simulink model "UsvNuFLController"  (R2019b)
settings: Solver=ode3  StartTime=0.0  StopTime=Inf  FixedStep=0.01  RelTol=1e-3  EnableMultiTasking=on
undefined symbols (not defined in the file): Theta, X
libraries: robotlib x8, simulink x2
settings Model: Creator=The MathWorks, Inc.  LastModifiedBy=alex
settings DataIOCC: LimitDataPoints=on  SaveFormat=Array  ReturnWorkspaceOutputs=off
settings OptimizationCC: LifeSpan=Inf  MaxStackSize=64
settings DebuggingCC: SolverPrmCheckMsg=warning  AllowSymbolicDim=off  SFUnexpectedBacktrackingDiag=warning  SFNoUnconditionalDefaultTransitionDiag=warning  SFExecutionAtInitializationDiag=none  ArithmeticOperatorsInVariantConditions=warning
settings HardwareCC: ProdBitPerLong=64  ProdHWDeviceType=Intel->x86-64 (Linux 64)  TargetHWDeviceType=Generic->Unspecified (assume 32-bit Generic)  UseEmbeddedCoderFeatures=off
settings ModelReferenceCC: PropagateSignalLabelsOutOfModel=off
settings SFSimCC: SimUseLocalCustomCode=off  CustomCodeUndefinedFunction=UseInterfaceOnly
settings RTWCC: SystemTargetFile=ert.tlc  HardwareBoard=Robot Operating System (ROS)  TemplateMakefile=ert_default_tmf  RTWUseLocalCustomCode=off  Toolchain=Catkin  TargetLang=C++
settings CodeAppCC: StateflowObjectComments=on
settings ERTTargetCC: MultiwordLength=2048  ERTCustomFileBanners=off  MultiInstanceERTCode=on  CodeInterfacePackaging=C++ class  SupportContinuousTime=on  SupportNonInlinedSFcns=on  RemoveResetFunc=off  SupportVariableSizeSignals=on  ModelStepFunctionPrototypeControlCompliant=off  RootIOFormat=Structure reference  ConvertIfToSwitch=off  SuppressUnreachableDefaultCases=off
settings ConfigComp: CovMetricSettings=dw  CovHtmlReporting=on  CovSaveCumulativeToWorkspaceVar=on  CovSaveSingleToWorkspaceVar=on  CovExternalEMLEnable=off  CovSFcnEnable=off

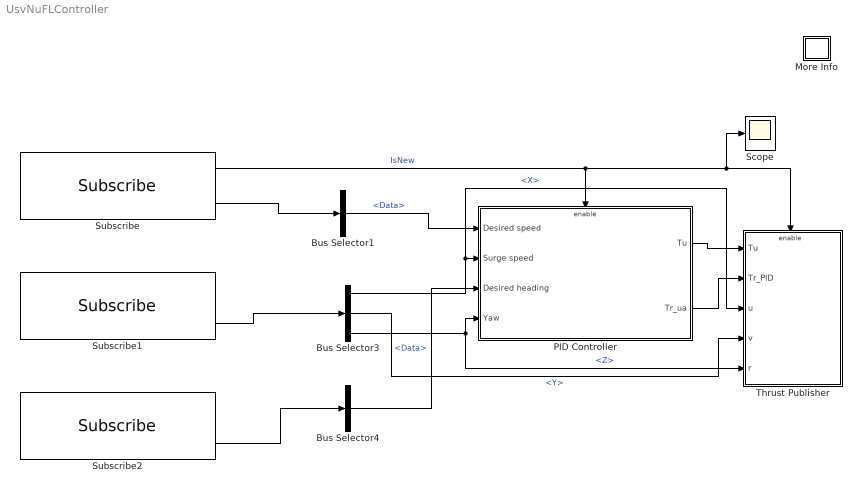
== system UsvNuFLController ==
  Bus Selector1 : BusSelector  OutputSignals=Data
  Bus Selector3 : BusSelector  OutputSignals=X,Y,Z
  Bus Selector4 : BusSelector  OutputSignals=Data
  More Info : Subsystem
      settings: OpenFcn=showdemo(bdroot(gcb))
      mask Display: disp('?')
  "PID Controller " : Subsystem
  Scope : Scope
  Subscribe : robotlib/Subscribe  topicSource=Select from ROS network  topic=/guidance/desired_speed  messageType=std_msgs/Float64  sampleTime=-1  messageQueueLength=51
      settings: SourceProductName=ROS Toolbox
  Subscribe1 : robotlib/Subscribe  topicSource=Select from ROS network  topic=/vectornav/ins_2d/local_vel  messageType=geometry_msgs/Vector3  sampleTime=-1  messageQueueLength=51
      settings: SourceProductName=ROS Toolbox
  Subscribe2 : robotlib/Subscribe  topicSource=Select from ROS network  topic=/guidance/desired_heading  messageType=std_msgs/Float64  sampleTime=-1  messageQueueLength=51
      settings: SourceProductName=ROS Toolbox
  Thrust Publisher : Subsystem
  wires:
  Subscribe/2 -> Bus Selector1/1
  Bus Selector1/1 -> "PID Controller "/1(Desired speed)  "<Data>"
  "PID Controller "/1(Tu) -> Thrust Publisher/1(Tu)
  Subscribe/1 -> Thrust Publisher/Enable, Scope/1, "PID Controller "/Enable  "IsNew"
  Subscribe1/2 -> Bus Selector3/1
  Bus Selector3/1 -> Thrust Publisher/3(u), "PID Controller "/2(Surge speed)  "<X>"
  Subscribe2/2 -> Bus Selector4/1
  Bus Selector4/1 -> "PID Controller "/3(Desired heading)  "<Data>"
  "PID Controller "/2(Tr_ua) -> Thrust Publisher/2(Tr_PID)
  Bus Selector3/3 -> "PID Controller "/4(Yaw), Thrust Publisher/5(r)  "<Z>"
  Bus Selector3/2 -> Thrust Publisher/4(v)  "<Y>"

== system UsvNuFLController/More Info ==

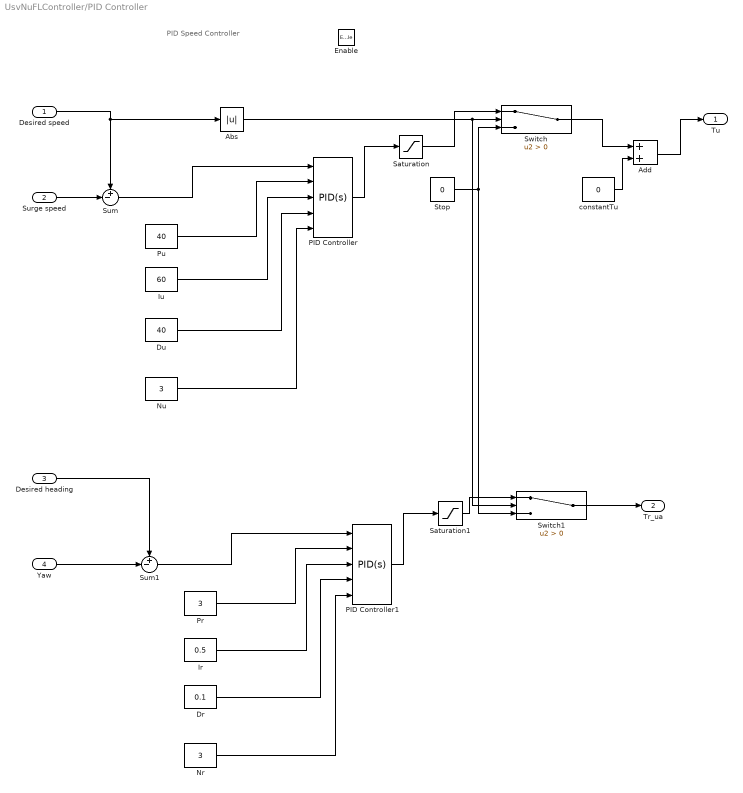
== system UsvNuFLController/PID Controller  ==
  note: PID Speed Controller
  Desired speed : Inport
  Surge speed : Inport  Port=2
  Desired heading : Inport  Port=3
  Yaw : Inport  Port=4
  Enable : EnablePort
  Abs : Abs
  Add : Sum
  Dr : Constant  Value=0.1
  Du : Constant  Value=40
  Ir : Constant  Value=0.5
  Iu : Constant  Value=60
  Nr : Constant  Value=3
  Nu : Constant  Value=3
  PID Controller : simulink/Continuous/PID Controller  Controller=PID  Form=Parallel  TimeDomain=Continuous-time  SampleTime=-1  IntegratorMethod=Forward Euler  FilterMethod=Forward Euler  ControllerParametersSource=external  P=1  I=1  D=0  UseFilter=on  N=100  TunerSelectOption=Transfer Function Based (PID Tuner App)  InitialConditionSource=internal  InitialConditionForIntegrator=0  InitialConditionForFilter=0  DifferentiatorICPrevScaledInput=0  ExternalReset=none  TrackingMode=off  Kt=1  LimitOutput=off  UpperSaturationLimit=inf  LowerSaturationLimit=-inf  LinearizeAsGain=on  AntiWindupMode=none  Kb=1  POutMin=[]  POutMax=[]  IOutMin=[]  IOutMax=[]  DOutMin=[]  DOutMax=[]  NOutMin=[]  NOutMax=[]  SumOutMin=[]  SumOutMax=[]  SaturationOutMin=[]  SaturationOutMax=[]  PParamMin=[]  PParamMax=[]  IParamMin=[]  IParamMax=[]  DParamMin=[]  DParamMax=[]  NParamMin=[]  NParamMax=[]  KbParamMin=[]  KbParamMax=[]  KtParamMin=[]  KtParamMax=[]  KbOutMin=[]  KbOutMax=[]  KtOutMin=[]  KtOutMax=[]  IntegratorOutMin=[]  IntegratorOutMax=[]  FilterOutMin=[]  FilterOutMax=[]  SumI1OutMin=[]  SumI1OutMax=[]  SumI2OutMin=[]  SumI2OutMax=[]  SumI3OutMin=[]  SumI3OutMax=[]  SumI4OutMin=[]  SumI4OutMax=[]  SumDOutMin=[]  SumDOutMax=[]  DifferentiatorOutMin=[]  DifferentiatorOutMax=[]  FilterDiffOutCoefMin=[]  FilterDiffOutCoefMax=[]  ReciprocalOutMin=[]  ReciprocalOutMax=[]  SumDenOutMin=[]  SumDenOutMax=[]  SumNumOutMin=[]  SumNumOutMax=[]  DivideOutMin=[]  DivideOutMax=[]  IntegratorContinuousStateAttributes=''  IntegratorStateMustResolveToSignalObject=off  IntegratorRTWStateStorageClass=Auto  FilterContinuousStateAttributes=''  FilterStateMustResolveToSignalObject=off  FilterRTWStateStorageClass=Auto  ParallelPVariant=ExternalParameters  IdealPVariant=Disabled  IVariant=ExternalParameters  DVariant=ExternalParameters  IntegratorVariant=Continuous  SatVariant=Disabled  AWVariant=Passthrough  PCopyVariant=Disabled  TRVariant=Disabled  FdbkBlocksVariant=Forward  IdealPFdbkVariant=Disabled  SatFdbkVariant=Disabled  DerivativeFilterVariant=ContFilter  NVariant=ExternalParameters  NCopyVariant=Disabled  FilterICVariant=InternalICsFilter  IntegratorICVariant=InternalICs  ExternalResetVariant=Disabled  TRSumVariant=Passthrough  SumFdbkVariant=Disabled  SumVariant=Sum_PID
  PID Controller1 : simulink/Continuous/PID Controller  Controller=PID  Form=Parallel  TimeDomain=Continuous-time  SampleTime=-1  IntegratorMethod=Forward Euler  FilterMethod=Forward Euler  ControllerParametersSource=external  P=1  I=1  D=0  UseFilter=on  N=100  TunerSelectOption=Transfer Function Based (PID Tuner App)  InitialConditionSource=internal  InitialConditionForIntegrator=0  InitialConditionForFilter=0  DifferentiatorICPrevScaledInput=0  ExternalReset=none  TrackingMode=off  Kt=1  LimitOutput=off  UpperSaturationLimit=inf  LowerSaturationLimit=-inf  LinearizeAsGain=on  AntiWindupMode=none  Kb=1  POutMin=[]  POutMax=[]  IOutMin=[]  IOutMax=[]  DOutMin=[]  DOutMax=[]  NOutMin=[]  NOutMax=[]  SumOutMin=[]  SumOutMax=[]  SaturationOutMin=[]  SaturationOutMax=[]  PParamMin=[]  PParamMax=[]  IParamMin=[]  IParamMax=[]  DParamMin=[]  DParamMax=[]  NParamMin=[]  NParamMax=[]  KbParamMin=[]  KbParamMax=[]  KtParamMin=[]  KtParamMax=[]  KbOutMin=[]  KbOutMax=[]  KtOutMin=[]  KtOutMax=[]  IntegratorOutMin=[]  IntegratorOutMax=[]  FilterOutMin=[]  FilterOutMax=[]  SumI1OutMin=[]  SumI1OutMax=[]  SumI2OutMin=[]  SumI2OutMax=[]  SumI3OutMin=[]  SumI3OutMax=[]  SumI4OutMin=[]  SumI4OutMax=[]  SumDOutMin=[]  SumDOutMax=[]  DifferentiatorOutMin=[]  DifferentiatorOutMax=[]  FilterDiffOutCoefMin=[]  FilterDiffOutCoefMax=[]  ReciprocalOutMin=[]  ReciprocalOutMax=[]  SumDenOutMin=[]  SumDenOutMax=[]  SumNumOutMin=[]  SumNumOutMax=[]  DivideOutMin=[]  DivideOutMax=[]  IntegratorContinuousStateAttributes=''  IntegratorStateMustResolveToSignalObject=off  IntegratorRTWStateStorageClass=Auto  FilterContinuousStateAttributes=''  FilterStateMustResolveToSignalObject=off  FilterRTWStateStorageClass=Auto  ParallelPVariant=ExternalParameters  IdealPVariant=Disabled  IVariant=ExternalParameters  DVariant=ExternalParameters  IntegratorVariant=Continuous  SatVariant=Disabled  AWVariant=Passthrough  PCopyVariant=Disabled  TRVariant=Disabled  FdbkBlocksVariant=Forward  IdealPFdbkVariant=Disabled  SatFdbkVariant=Disabled  DerivativeFilterVariant=ContFilter  NVariant=ExternalParameters  NCopyVariant=Disabled  FilterICVariant=InternalICsFilter  IntegratorICVariant=InternalICs  ExternalResetVariant=Disabled  TRSumVariant=Passthrough  SumFdbkVariant=Disabled  SumVariant=Sum_PID
  Pr : Constant  Value=3
  Pu : Constant  Value=40
  Saturation : Saturate  UpperLimit=73  LowerLimit=-60
  Saturation1 : Saturate  UpperLimit=14  LowerLimit=-14
  Stop : Constant  Value=0
  Sum : Sum  Inputs=+-|
  Sum1 : Sum  Inputs=+-|
  Switch : Switch  Criteria=u2 > Threshold
  Switch1 : Switch  Criteria=u2 > Threshold
  constantTu : Constant  Value=0
  Tu : Outport  VectorParamsAs1DForOutWhenUnconnected=off
  Tr_ua : Outport  Port=2  VectorParamsAs1DForOutWhenUnconnected=off
  wires:
  Desired speed/1 -> Abs/1, Sum/1
  Surge speed/1 -> Sum/2
  Pu/1 -> PID Controller/2
  Stop/1 -> Switch1/3, Switch/3
  Switch/1 -> Add/1
  Sum/1 -> PID Controller/1
  Iu/1 -> PID Controller/3
  PID Controller/1 -> Saturation/1
  Saturation/1 -> Switch/1
  Du/1 -> PID Controller/4
  Nu/1 -> PID Controller/5
  Abs/1 -> Switch1/2, Switch/2
  Nr/1 -> PID Controller1/5
  Desired heading/1 -> Sum1/1
  Dr/1 -> PID Controller1/4
  PID Controller1/1 -> Saturation1/1
  Ir/1 -> PID Controller1/3
  Yaw/1 -> Sum1/2
  Saturation1/1 -> Switch1/1
  Pr/1 -> PID Controller1/2
  Sum1/1 -> PID Controller1/1
  Switch1/1 -> Tr_ua/1
  constantTu/1 -> Add/2
  Add/1 -> Tu/1

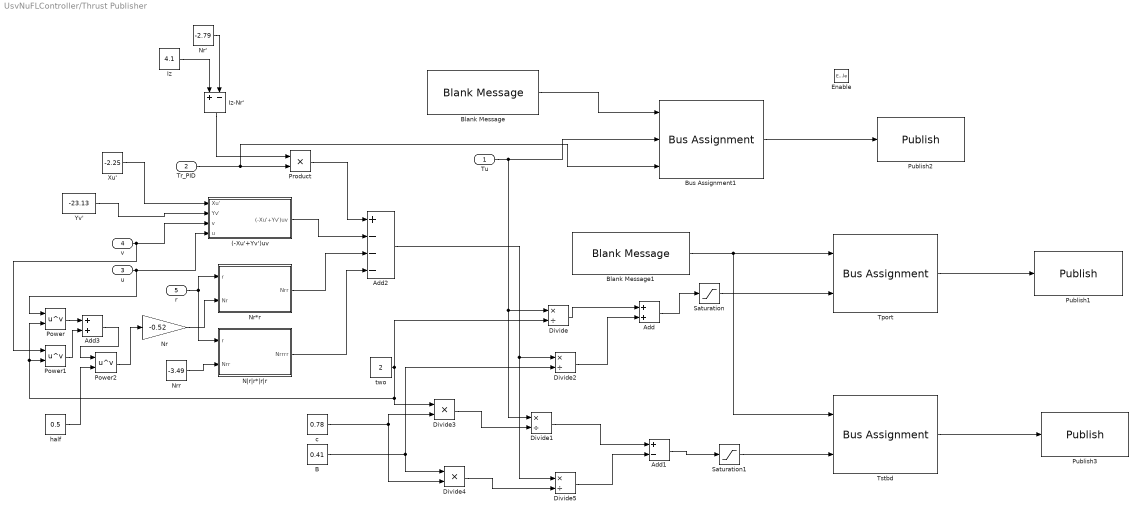
== system UsvNuFLController/Thrust Publisher ==
  Tu : Inport
  Tr_PID : Inport  Port=2
  u : Inport  Port=3
  v : Inport  Port=4
  r : Inport  Port=5
  Enable : EnablePort
  (-Xu'+Yv')uv : Subsystem
  Add : Sum
  Add1 : Sum  Inputs=+-
  Add2 : Sum  Inputs=+---
  Add3 : Sum
  B : Constant  Value=0.41
  Blank Message : robotlib/Blank Message  messageClass=Message  entityType=geometry_msgs/Pose2D  messageType=geometry_msgs/Pose2D  SampleTime=inf
      settings: SourceProductName=ROS Toolbox
  Blank Message1 : robotlib/Blank Message  messageClass=Message  entityType=std_msgs/Float64  messageType=std_msgs/Float64  SampleTime=inf
      settings: SourceProductName=ROS Toolbox
  Bus Assignment1 : BusAssignment  DialogController=Simulink.DDGSource_BusAssignment  AssignedSignals=X,Theta
  Divide{,1..2,5} (4 alike) : Product  Inputs=*/
  Divide3 : Product  Inputs=**
  Divide4 : Product  Inputs=**
  "Iz " : Constant  Value=4.1
  Iz-Nr' : Sum  Inputs=+-
  Nr : Gain  Gain=-0.52
  Nr' : Constant  Value=-2.79
  Nr*r : Subsystem
  Nrr : Constant  Value=-3.49
  N|r|r*|r|r : Subsystem
  Power : Math  Operator=pow  SignedPower=off  SaturateOnIntegerOverflow=on
  Power1 : Math  Operator=pow  SignedPower=off  SaturateOnIntegerOverflow=on
  Power2 : Math  Operator=pow  SignedPower=off  SaturateOnIntegerOverflow=on
  Product : Product
  Publish1 : robotlib/Publish  topicSource=Select from ROS network  topic=/usv_control/controller/left_thruster  messageType=std_msgs/Float64  messageQueueLength=105
      settings: SourceProductName=ROS Toolbox
  Publish2 : robotlib/Publish  topicSource=Select from ROS network  topic=/usv_control/controller/control_input  messageType=geometry_msgs/Pose2D  messageQueueLength=105
      settings: SourceProductName=ROS Toolbox
  Publish3 : robotlib/Publish  topicSource=Select from ROS network  topic=/usv_control/controller/right_thruster  messageType=std_msgs/Float64  messageQueueLength=105
      settings: SourceProductName=ROS Toolbox
  Saturation : Saturate  UpperLimit=36.5  LowerLimit=-30
  Saturation1 : Saturate  UpperLimit=36.5  LowerLimit=-30
  Tport : BusAssignment  DialogController=Simulink.DDGSource_BusAssignment  AssignedSignals=Data
  Tstbd : BusAssignment  DialogController=Simulink.DDGSource_BusAssignment  AssignedSignals=Data
  Xu' : Constant  Value=-2.25
  Yv' : Constant  Value=-23.13
  c : Constant  Value=0.78
  half : Constant  Value=0.5
  two : Constant  Value=2
  wires:
  Bus Assignment1/1 -> Publish2/1
  Blank Message/1 -> Bus Assignment1/1
  Tu/1 -> Bus Assignment1/2, Divide1/1, Divide/1
  Tport/1 -> Publish1/1
  Tstbd/1 -> Publish3/1
  Blank Message1/1 -> Tstbd/1, Tport/1
  two/1 -> Power1/2, Power/2, Divide3/1, Divide/2
  Saturation/1 -> Tport/2
  Saturation1/1 -> Tstbd/2
  Add2/1 -> Divide2/1, Divide5/1
  Divide/1 -> Add/1
  B/1 -> Divide4/1, Divide2/2
  Divide2/1 -> Add/2
  Add/1 -> Saturation/1
  c/1 -> Divide3/2, Divide4/2
  Add1/1 -> Saturation1/1
  Divide3/1 -> Divide1/2
  Divide4/1 -> Divide5/2
  Divide1/1 -> Add1/1
  Divide5/1 -> Add1/2
  Yv'/1 -> (-Xu'+Yv')uv/2(Yv')
  (-Xu'+Yv')uv/1((-Xu'+Yv')uv) -> Add2/2
  Tr_PID/1 -> Bus Assignment1/3, Product/2
  Nr/1 -> Nr*r/2(Nr)
  v/1 -> Power1/1, (-Xu'+Yv')uv/3(v)
  Product/1 -> Add2/1
  "Iz "/1 -> Iz-Nr'/1
  u/1 -> Power/1, (-Xu'+Yv')uv/4(u)
  Nr*r/1(Nrr) -> Add2/3
  Iz-Nr'/1 -> Product/1
  r/1 -> N|r|r*|r|r/1(r), Nr*r/1(r)
  Nr'/1 -> Iz-Nr'/2
  Xu'/1 -> (-Xu'+Yv')uv/1(Xu')
  Power/1 -> Add3/1
  Add3/1 -> Power2/1
  half/1 -> Power2/2
  Power2/1 -> Nr/1
  Power1/1 -> Add3/2
  Nrr/1 -> N|r|r*|r|r/2(Nrr)
  N|r|r*|r|r/1(Nrrrr) -> Add2/4

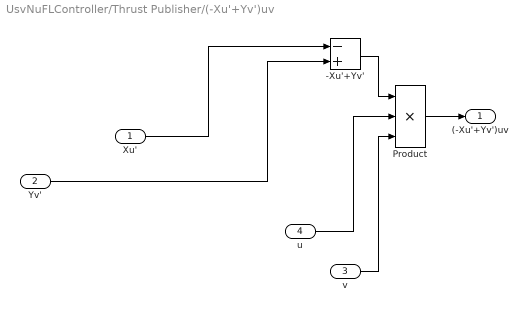
== system UsvNuFLController/Thrust Publisher/(-Xu'+Yv')uv ==
  Xu' : Inport
  Yv' : Inport  Port=2
  v : Inport  Port=3
  u : Inport  Port=4
  -Xu'+Yv' : Sum  Inputs=-+
  Product : Product  Inputs=3
  (-Xu'+Yv')uv : Outport  VectorParamsAs1DForOutWhenUnconnected=off
  wires:
  Yv'/1 -> -Xu'+Yv'/2
  v/1 -> Product/3
  -Xu'+Yv'/1 -> Product/1
  u/1 -> Product/2
  Product/1 -> (-Xu'+Yv')uv/1
  Xu'/1 -> -Xu'+Yv'/1

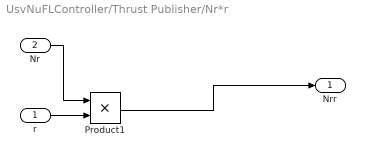
== system UsvNuFLController/Thrust Publisher/Nr*r ==
  r : Inport
  Nr : Inport  Port=2
  Product1 : Product
  Nrr : Outport  VectorParamsAs1DForOutWhenUnconnected=off
  wires:
  Product1/1 -> Nrr/1
  Nr/1 -> Product1/1
  r/1 -> Product1/2

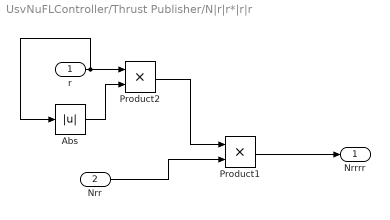
== system UsvNuFLController/Thrust Publisher/N|r|r*|r|r ==
  r : Inport
  Nrr : Inport  Port=2
  Abs : Abs
  Product1 : Product
  Product2 : Product
  Nrrrr : Outport  VectorParamsAs1DForOutWhenUnconnected=off
  wires:
  Product1/1 -> Nrrrr/1
  r/1 -> Abs/1, Product2/1
  Abs/1 -> Product2/2
  Nrr/1 -> Product1/2
  Product2/1 -> Product1/1
